simulink model "MotorMuestreado"  (R2017a)
settings: Solver=VariableStepAuto  StartTime=0.0  StopTime=1.0  RelTol=1e-3
values from neighbouring files (symbols this model uses):
  b = 1.1    [Continuo.m]    (also in Discreto.m)
  J = 15    [Continuo.m]    (also in Discreto.m)
  K = 6.69    [Continuo.m]    (also in Discreto.m)
  L = 0.00279    [Continuo.m]    (also in Discreto.m)
  R = 0.051    [Continuo.m]    (also in Discreto.m)
settings Model: Creator=joaqu  LastModifiedBy=joaqu

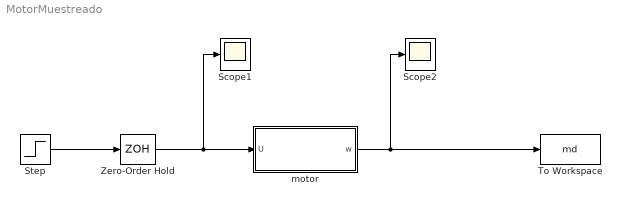
== system MotorMuestreado ==
  Scope1 : Scope
  Scope2 : Scope
  Step : Step  Time=0  After=440  SampleTime=0
  To Workspace : ToWorkspace  VariableName=md  SaveFormat=Timeseries  SampleTime=-1
  Zero-Order Hold : ZeroOrderHold  SampleTime=-1
  "motor " : Subsystem
  wires:
  Zero-Order Hold/1 -> Scope1/1, "motor "/1(U)
  "motor "/1(w) -> To Workspace/1, Scope2/1
  Step/1 -> Zero-Order Hold/1

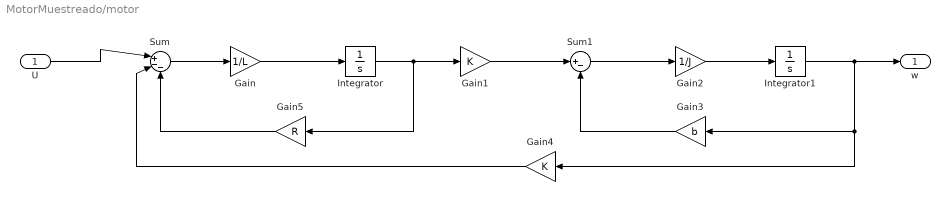
== system MotorMuestreado/motor  ==
  U : Inport
  Gain : Gain  Gain=1/L
  Gain1 : Gain  Gain=K
  Gain2 : Gain  Gain=1/J
  Gain3 : Gain  Gain=b
  Gain4 : Gain  Gain=K
  Gain5 : Gain  Gain=R
  Integrator : Integrator
  Integrator1 : Integrator
  Sum : Sum  Inputs=|+--
  Sum1 : Sum  Inputs=|+-
  w : Outport
  wires:
  Gain4/1 -> Sum/2
  Gain1/1 -> Sum1/1
  Gain5/1 -> Sum/3
  Integrator/1 -> Gain5/1, Gain1/1
  Gain3/1 -> Sum1/2
  Sum1/1 -> Gain2/1
  U/1 -> Sum/1
  Gain2/1 -> Integrator1/1
  Gain/1 -> Integrator/1
  Integrator1/1 -> w/1, Gain4/1, Gain3/1
  Sum/1 -> Gain/1
